simulink model "task1_simulink"  (R2023a)
settings: Solver=VariableStepAuto  StartTime=0.0  StopTime=10.0  RelTol=1e-3
libraries: cstblocks x8, simulink x4
settings Model: Creator=aalia  LastModifiedBy=aalia

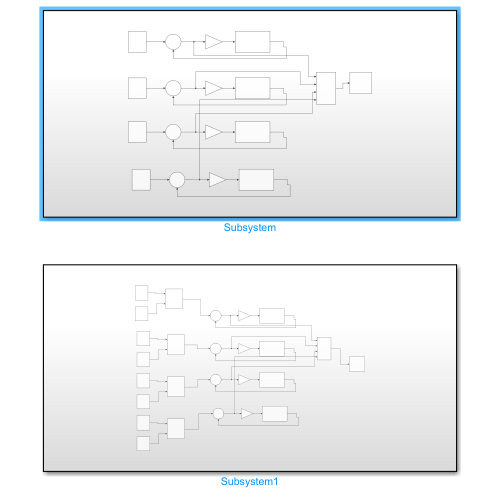
[thumbnail: Simulink's stored preview of the top-level diagram]
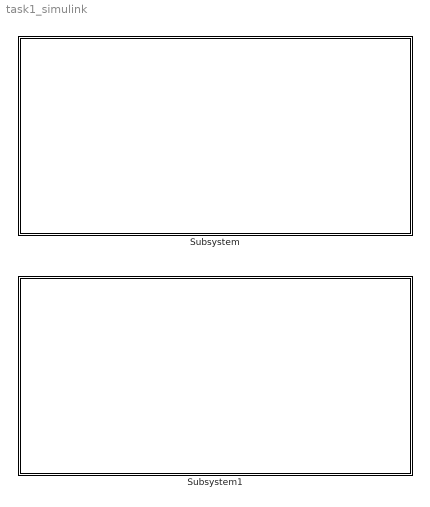
== system task1_simulink ==
  Subsystem : Subsystem
  Subsystem1 : Subsystem

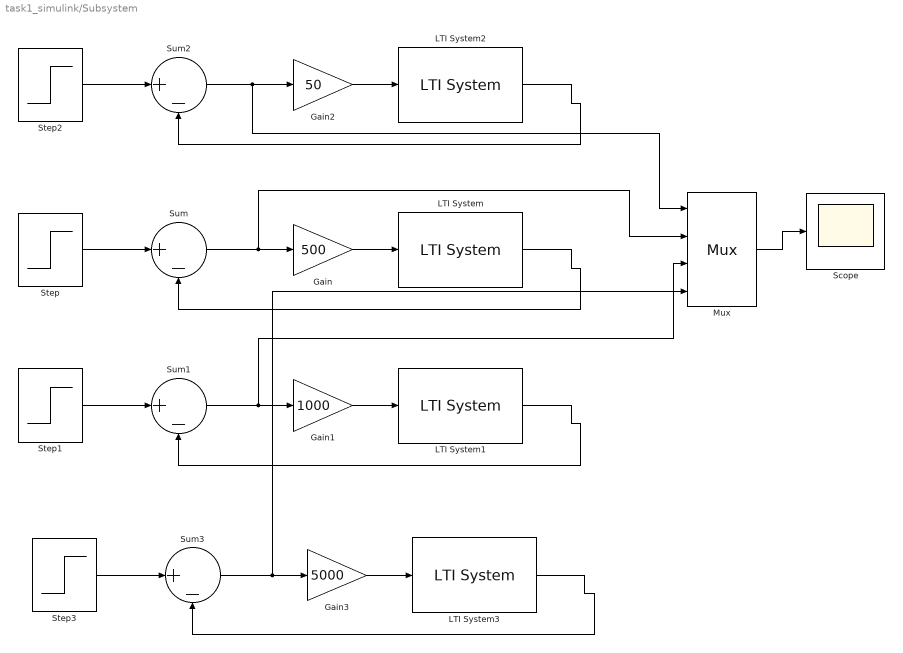
== system task1_simulink/Subsystem ==
  Gain : Gain  Gain=500
  Gain1 : Gain  Gain=1000
  Gain2 : Gain  Gain=50
  Gain3 : Gain  Gain=5000
  LTI System : cstblocks/LTI System  sys=|  IC=[]
      | tf([1 6],[1 32 367 1776 3024
      | ])
  LTI System1 : cstblocks/LTI System  sys=|  IC=[]
      | tf([1 6],[1 32 367 1776 3024
      | ])
  LTI System2 : cstblocks/LTI System  sys=|  IC=[]
      | tf([1 6],[1 32 367 1776 3024
      | ])
  LTI System3 : cstblocks/LTI System  sys=|  IC=[]
      | tf([1 6],[1 32 367 1776 3024
      | ])
  Mux : Mux
  Scope : Scope
  Step{,1..3} (4 alike) : Step  Time=0  After=5  SampleTime=0
  Sum{,1..3} (4 alike) : Sum  Inputs=|+-
  wires:
  Sum2/1 -> Mux/1, Gain2/1
  Gain2/1 -> LTI System2/1
  Step3/1 -> Sum3/1
  Sum1/1 -> Mux/3, Gain1/1
  Sum/1 -> Mux/2, Gain/1
  Gain/1 -> LTI System/1
  Step/1 -> Sum/1
  Sum3/1 -> Mux/4, Gain3/1
  Step1/1 -> Sum1/1
  Mux/1 -> Scope/1
  LTI System/1 -> Sum/2
  LTI System1/1 -> Sum1/2
  Gain1/1 -> LTI System1/1
  Step2/1 -> Sum2/1
  LTI System2/1 -> Sum2/2
  LTI System3/1 -> Sum3/2
  Gain3/1 -> LTI System3/1

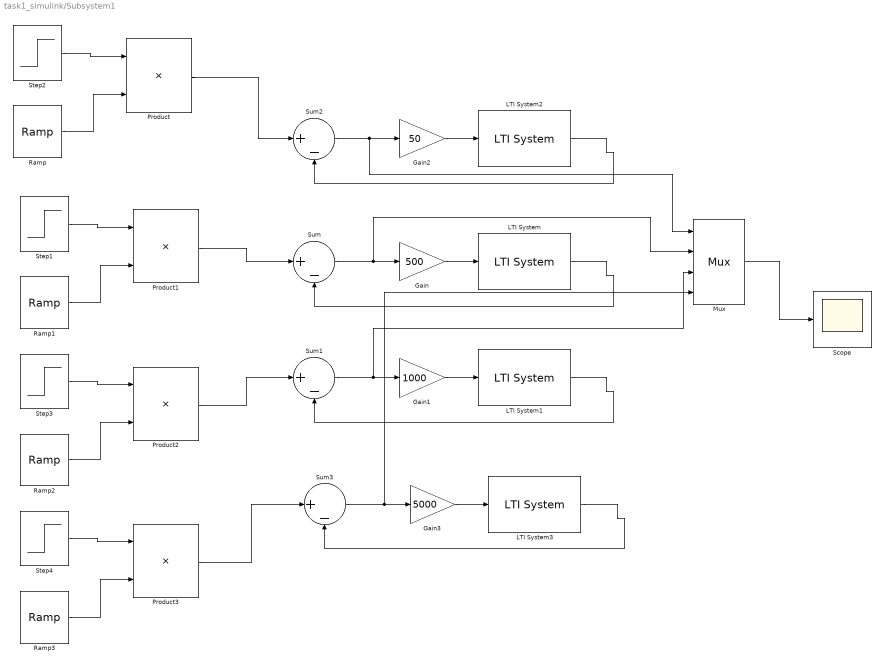
== system task1_simulink/Subsystem1 ==
  Gain : Gain  Gain=500
  Gain1 : Gain  Gain=1000
  Gain2 : Gain  Gain=50
  Gain3 : Gain  Gain=5000
  LTI System : cstblocks/LTI System  sys=|  IC=[]
      | tf([1 6],[1 32 367 1776 3024
      | ])
  LTI System1 : cstblocks/LTI System  sys=|  IC=[]
      | tf([1 6],[1 32 367 1776 3024
      | ])
  LTI System2 : cstblocks/LTI System  sys=|  IC=[]
      | tf([1 6],[1 32 367 1776 3024
      | ])
  LTI System3 : cstblocks/LTI System  sys=|  IC=[]
      | tf([1 6],[1 32 367 1776 3024
      | ])
  Mux : Mux
  Product{,1..3} (4 alike) : Product
  Ramp{,1..3} (4 alike) : simulink/Sources/Ramp  slope=1  start=0  InitialOutput=0
  Scope : Scope
  Step{1..4} (4 alike) : Step  Time=0  After=5  SampleTime=0
  Sum{,1..3} (4 alike) : Sum  Inputs=|+-
  wires:
  Sum2/1 -> Mux/1, Gain2/1
  Gain2/1 -> LTI System2/1
  Product3/1 -> Sum3/1
  Sum1/1 -> Mux/3, Gain1/1
  Sum/1 -> Mux/2, Gain/1
  Gain/1 -> LTI System/1
  Product1/1 -> Sum/1
  Sum3/1 -> Mux/4, Gain3/1
  Product2/1 -> Sum1/1
  LTI System/1 -> Sum/2
  LTI System1/1 -> Sum1/2
  Gain1/1 -> LTI System1/1
  LTI System2/1 -> Sum2/2
  LTI System3/1 -> Sum3/2
  Gain3/1 -> LTI System3/1
  Product/1 -> Sum2/1
  Step2/1 -> Product/1
  Ramp/1 -> Product/2
  Step1/1 -> Product1/1
  Ramp1/1 -> Product1/2
  Step3/1 -> Product2/1
  Ramp2/1 -> Product2/2
  Step4/1 -> Product3/1
  Ramp3/1 -> Product3/2
  Mux/1 -> Scope/1
